simulink model "RC_Circuit_Inverters_Charge"  (R2017b)
settings: Solver=VariableStepAuto  StartTime=0.0  StopTime=20  RelTol=1e-3
libraries: fl_lib x6, nesl_utility x3, simulink x2
settings Model: Creator=cspt  LastModifiedBy=cspt

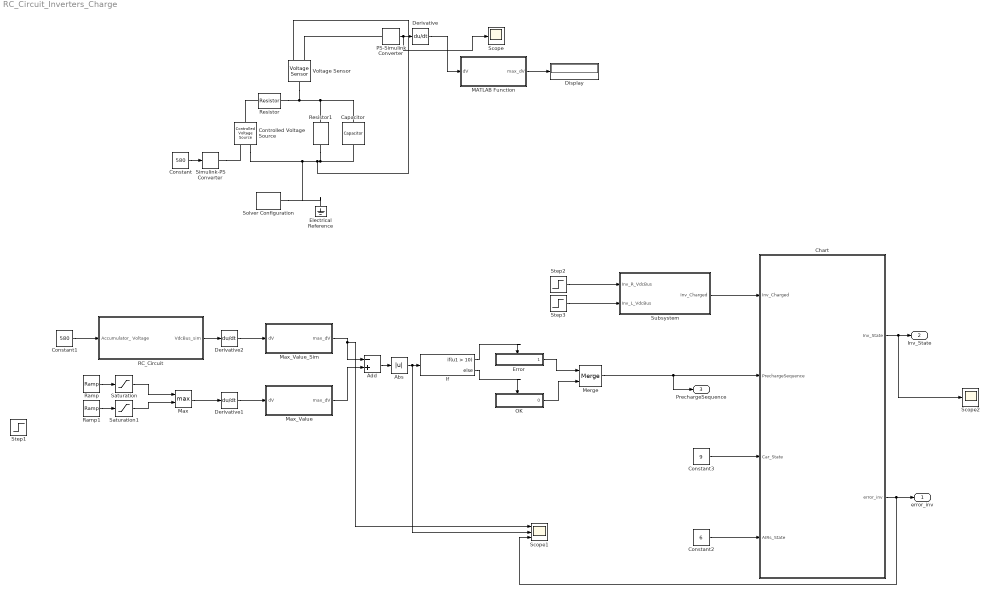
== system RC_Circuit_Inverters_Charge ==
  Abs : Abs
  Add : Sum  Inputs=-+
  Capacitor : fl_lib/Electrical/Electrical Elements/Capacitor  c=640e-6 F  r=1e-6 Ohm  g=0 1/Ohm  i_specify=off  i_priority=None  i=0 A  i_nominal_specify=off  i_nominal_unit=A  i_nominal_value=1  v_specify=off  v_priority=None  v=0 V  v_nominal_specify=off  v_nominal_unit=V  v_nominal_value=1  vc_specify=off  vc_priority=High  vc=0 V  vc_nominal_specify=off  vc_nominal_unit=V  vc_nominal_value=1
  Chart : Stateflow chart  TreatAsAtomicUnit=on
  Constant : Constant  Value=580
  Constant1 : Constant  Value=580
  Constant2 : Constant  Value=6
  Constant3 : Constant  Value=9
  Controlled Voltage Source : fl_lib/Electrical/Electrical Sources/Controlled Voltage Source
  Derivative : Derivative
  Derivative1 : Derivative
  Derivative2 : Derivative
  Display : Display
  Electrical Reference : fl_lib/Electrical/Electrical Elements/Electrical Reference
  Error : Subsystem  TreatAsAtomicUnit=on
  If : If  IfExpression=u1 > 10
  MATLAB Function : MATLAB Function  TreatAsAtomicUnit=on
  Max : MinMax  Function=max  Inputs=2
  Max_Value : MATLAB Function  TreatAsAtomicUnit=on
  Max_Value_Sim : MATLAB Function  TreatAsAtomicUnit=on
  Merge : Merge
  OK : Subsystem  TreatAsAtomicUnit=on
  PS-Simulink Converter : nesl_utility/PS-Simulink Converter  PhysicalDomain=network_engine_domain  SubClassName=ps_output  LeftPortType=input  RightPortType=output  PseudoPeriodic=off  Frequencies=[]  Unit=1  AffineConversion=off
  RC_Circuit : Subsystem
  Ramp : simulink/Sources/Ramp  slope=580  start=0  X0=0
  Ramp1 : simulink/Sources/Ramp  slope=580  start=0  X0=0
  Resistor : fl_lib/Electrical/Electrical Elements/Resistor  R=470 Ohm  i_specify=off  i_priority=None  i=0 A  i_nominal_specify=off  i_nominal_unit=A  i_nominal_value=1  v_specify=off  v_priority=None  v=0 V  v_nominal_specify=off  v_nominal_unit=V  v_nominal_value=1
  Resistor1 : fl_lib/Electrical/Electrical Elements/Resistor  R=25000 Ohm  i_specify=off  i_priority=None  i=0 A  i_nominal_specify=off  i_nominal_unit=A  i_nominal_value=1  v_specify=off  v_priority=None  v=0 V  v_nominal_specify=off  v_nominal_unit=V  v_nominal_value=1
  Saturation : Saturate  UpperLimit=580  LowerLimit=0
  Saturation1 : Saturate  UpperLimit=580  LowerLimit=0
  Scope : Scope
  Scope1 : Scope  NumInputPorts=3
  Scope2 : Scope
  Simulink-PS Converter : nesl_utility/Simulink-PS Converter  PhysicalDomain=network_engine_domain  SubClassName=ps_input  LeftPortType=input  RightPortType=output  PseudoPeriodic=off  Frequencies=[]  NoiseDistribution=none  NoiseParameters=[]  Unit=1  AffineConversion=off  FilteringAndDerivatives=provide  SimscapeFilterOrder=1  InputFilterTimeConstant=0.001  UdotUserProvided=0
  Solver Configuration : nesl_utility/Solver Configuration  PhysicalDomain=network_engine_domain  SubClassName=solver  LeftPortType=input  RightPortType=generic  Accelerate=off  Tones=[]  Harmonics=[]  SimulateNoise=off  Profile=off  UseLocalSampling=off  EnableSwitchedLinearOptims=on  FrequencyDomain=off  UseCCode=off  RelTol=0.001  AbsTol=1e-06  MinStep=1e-09  ToWorkspace=off  RevertToSquareIcSolve=off  NumHomotopyIterations=100  PhasorMode=off  PhasorModeNumHarmonics=1  DoDC=off  ResidualTolerance=1e-09  UseLocalSolver=off  LocalSolverChoice=NE_BACKWARD_EULER_ADVANCER  LocalSolverSampleTime=0.001  DoFixedCost=off  MaxNonlinIter=3  MaxModeIter=2  LinearAlgebra=Sparse  DelaysMemoryBudget=1024  AutomaticFiltering=on  FilteringTimeConstant=0.001
  Step1 : Step  Time=0.5  After=580  SampleTime=0
  Step2 : Step  Time=5  After=580  SampleTime=0
  Step3 : Step  Time=5  After=580  SampleTime=0
  Subsystem : Subsystem
  Voltage Sensor : fl_lib/Electrical/Electrical Sensors/Voltage Sensor
  error_inv : Outport
  Inv_State : Outport  Port=2
  PrechargeSequence : Outport  Port=3
  wires:
  Constant/1 -> Simulink-PS Converter/1
  PS-Simulink Converter/1 -> Scope/1, Derivative/1
  Derivative/1 -> MATLAB Function/1(dV)
  MATLAB Function/1(max_dV) -> Display/1
  Step3/1 -> Subsystem/2(Inv_L_VdcBus)
  Constant3/1 -> Chart/3(Car_State)
  Max_Value/1(max_dV) -> Add/2
  RC_Circuit/1(VdcBus_sim) -> Derivative2/1
  Add/1 -> Abs/1
  Chart/2(error_inv) -> Scope1/3, error_inv/1
  Derivative1/1 -> Max_Value/1(dV)
  OK/1(0) -> Merge/2
  Error/1(1) -> Merge/1
  Max/1 -> Derivative1/1
  Merge/1 -> PrechargeSequence/1, Chart/2(PrechargeSequence)
  Max_Value_Sim/1(max_dV) -> Scope1/1, Add/1
  Ramp/1 -> Saturation/1
  Ramp1/1 -> Saturation1/1
  If/1 -> Error/Action
  Chart/1(Inv_State) -> Scope2/1, Inv_State/1
  Constant2/1 -> Chart/4(AIRs_State)
  Derivative2/1 -> Max_Value_Sim/1(dV)
  Step2/1 -> Subsystem/1(Inv_R_VdcBus)
  Constant1/1 -> RC_Circuit/1(Accumulator_ Voltage)
  Subsystem/1(Inv_Charged) -> Chart/1(Inv_Charged)
  If/2 -> OK/Action
  Saturation/1 -> Max/1
  Saturation1/1 -> Max/2
  Abs/1 -> Scope1/2, If/1
  connections:
  Resistor/RConn1 -- Voltage Sensor/LConn1 -- Resistor1/LConn1 -- Capacitor/LConn1
  Controlled Voltage Source/LConn1 -- Resistor/LConn1
  Controlled Voltage Source/RConn2 -- Electrical Reference/LConn1 -- Solver Configuration/RConn1 -- Voltage Sensor/RConn2 -- Resistor1/RConn1 -- Capacitor/RConn1
  PS-Simulink Converter/LConn1 -- Voltage Sensor/RConn1
  Simulink-PS Converter/RConn1 -- Controlled Voltage Source/RConn1

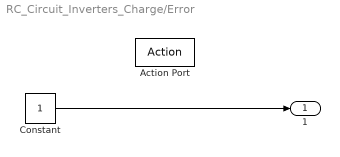
== system RC_Circuit_Inverters_Charge/Error ==
  Action Port : ActionPort  ActionType=then
  Constant : Constant
  1 : Outport
  wires:
  Constant/1 -> 1/1

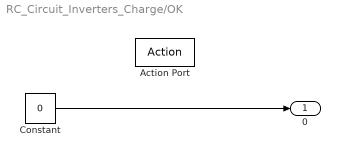
== system RC_Circuit_Inverters_Charge/OK ==
  Action Port : ActionPort  ActionType=else
  Constant : Constant  Value=0
  0 : Outport
  wires:
  Constant/1 -> 0/1

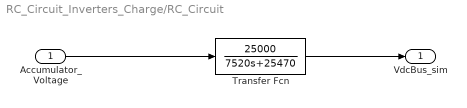
== system RC_Circuit_Inverters_Charge/RC_Circuit ==
  Accumulator_ Voltage : Inport
  Transfer Fcn : TransferFcn  Numerator=[25000]  Denominator=[7520 25470]
  VdcBus_sim : Outport
  wires:
  Accumulator_ Voltage/1 -> Transfer Fcn/1
  Transfer Fcn/1 -> VdcBus_sim/1

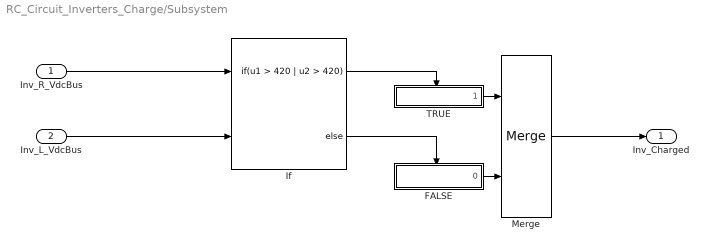
== system RC_Circuit_Inverters_Charge/Subsystem ==
  Inv_R_VdcBus : Inport
  Inv_L_VdcBus : Inport  Port=2
  FALSE : Subsystem  TreatAsAtomicUnit=on
  If : If  NumInputs=2  IfExpression=u1 > 420 | u2 > 420
  Merge : Merge
  TRUE : Subsystem  TreatAsAtomicUnit=on
  Inv_Charged : Outport
  wires:
  Inv_L_VdcBus/1 -> If/2
  Inv_R_VdcBus/1 -> If/1
  If/2 -> FALSE/Action
  Merge/1 -> Inv_Charged/1
  If/1 -> TRUE/Action
  TRUE/1(1) -> Merge/1
  FALSE/1(0) -> Merge/2

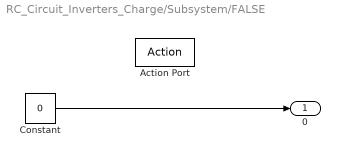
== system RC_Circuit_Inverters_Charge/Subsystem/FALSE ==
  Action Port : ActionPort  ActionType=else
  Constant : Constant  Value=0
  0 : Outport
  wires:
  Constant/1 -> 0/1

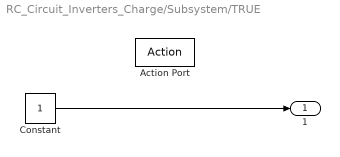
== system RC_Circuit_Inverters_Charge/Subsystem/TRUE ==
  Action Port : ActionPort  ActionType=then
  Constant : Constant
  1 : Outport
  wires:
  Constant/1 -> 1/1

== matlab function RC_Circuit_Inverters_Charge/Max_Value ==
  settings: updateMethod=DISCRETE
  data: dV input; max_dV output
function max_dV  = max_val(dV)

persistent dVpre

if isempty(dVpre)
    dVpre = 0;
end

if (dVpre > dV)
    max_dV = dVpre;
else
    max_dV = dV;
end
dVpre = max_dV;

== matlab function RC_Circuit_Inverters_Charge/MATLAB Function ==
  settings: updateMethod=DISCRETE
  data: dV input; max_dV output
function max_dV  = max_val(dV)

persistent dVpre

if isempty(dVpre)
    dVpre = 0;
end

if (dVpre > dV)
    max_dV = dVpre;
else
    max_dV = dV;
end
dVpre = max_dV;

== stateflow chart RC_Circuit_Inverters_Charge/Chart ==
  state InvDischarged
    entry: Inv_State = 0;
  state FAIL [group]
    state InvChargingError
      entry: Inv_State = 21;
    state OpenHVDBox
      entry: Inv_State = 24;
    InvChargingError -> OpenHVDBox : [AIRs_State == 0 & after(5, sec) & Inv_Charged == 1]{error_inv == 6}
  state InvCharging
    entry: Inv_State = 3;
  state InvCharged
    entry: Inv_State = 6;
  (default) -> InvDischarged : {error_inv=0}
  InvDischarged -> InvChargingError [order 2] : [AIRs_State == 6 & PrechargeSequence == 1]{error_inv==3}
  OpenHVDBox -> InvDischarged : [ Car_State == 0]
  InvDischarged -> InvCharging [order 1] : [AIRs_State == 6 & PrechargeSequence == 0]
  InvCharging -> InvChargingError [order 2] : [PrechargeSequence == 1 & Car_State == 9]
  InvCharging -> InvCharged [order 1] : [AIRs_State == 3 & Inv_Charged == 1 & PrechargeSequence == 0]
  InvCharged -> OpenHVDBox : [AIRs_State == 0 & after(5, sec) & Inv_Charged == 1]{error_inv == 6}
  data: Inv_Charged input; PrechargeSequence input; Car_State input; AIRs_State input; Inv_State output; error_inv output

== matlab function RC_Circuit_Inverters_Charge/Max_Value_Sim ==
  settings: updateMethod=DISCRETE
  data: dV input; max_dV output
function max_dV  = max_val(dV)

persistent dVpre

if isempty(dVpre)
    dVpre = 0;
end

if (dVpre > dV)
    max_dV = dVpre;
else
    max_dV = dV;
end
dVpre = max_dV;
